simulink model "MiniDAQ_FOSWEC_V3_Sim"  (R2020b)
settings: Solver=FixedStepAuto  StartTime=0.0  StopTime=inf  FixedStep=0.01  RelTol=1e-3
libraries: slrealtimeethercatlib x12
settings Model: SimulationMode=external  Creator=Bret  LastModifiedBy=Bret
settings SolverCC: ConcurrentTasks=on  PositivePriorityOrder=on
settings OptimizationCC: BlockReduction=off  OptimizeBlockIOStorage=off
settings HardwareCC: ProdBitPerLong=64  ProdLongLongMode=on  ProdHWDeviceType=Intel->x86-64 (Linux 64)
settings RTWCC: Description=Simulink Real-Time  SystemTargetFile=slrealtime.tlc  TemplateMakefile=slrealtime_default_tmf  Toolchain=Simulink Real-Time Toolchain  BuildConfiguration=Faster Runs  CodeExecutionProfiling=on  TargetLang=C++

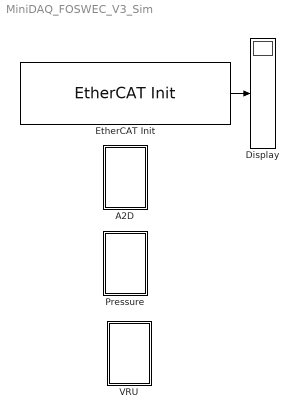
== system MiniDAQ_FOSWEC_V3_Sim ==
  A2D : Subsystem
  Display : Display
  EtherCAT Init : slrealtimeethercatlib/EtherCAT Init  Priority=0  config_file=C:\Users\Bret\Desktop\MiniDAQ_FOSWEC_V3\TwinCAT\MiniDAQ_V3.xml  device_id=0  pci_bus=0  pci_slot=0  pci_function=0  portnum=1  initstate=2  dctuning=0  enaDebug=0  enaDC=on  errLink=off  masterDbg=off  stateChgDbg=off  baseClock=off  masterCfg=off  logFile='c:\dbglog.txt'  sample_time=0.010000  DCMode=0
      settings: SourceProductBaseCode=XP
  Pressure : Subsystem
  VRU : Subsystem
  wires:
  EtherCAT Init/1 -> Display/1

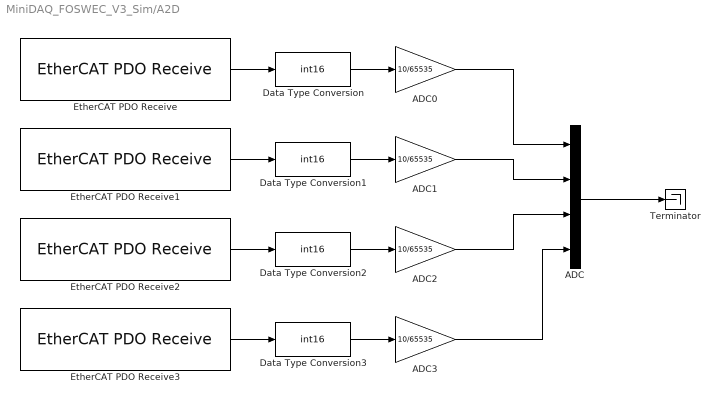
== system MiniDAQ_FOSWEC_V3_Sim/A2D ==
  ADC : Mux
  ADC{0..3} (4 alike) : Gain  Gain=10/65535
  Data Type Conversion{,1..3} (4 alike) : DataTypeConversion  OutDataTypeStr=int16
  EtherCAT PDO Receive : slrealtimeethercatlib/EtherCAT PDO Receive  Priority=2  sig_name=Box 1 (MiniDAQ_FOSWEC_V3).Inputs.ADC0  sig_offset=448  sig_type=uint16  type_size=16  sig_dim=1  device_id=0  sample_time=0.010000
      settings: SourceProductBaseCode=XP
  EtherCAT PDO Receive1 : slrealtimeethercatlib/EtherCAT PDO Receive  Priority=2  sig_name=Box 1 (MiniDAQ_FOSWEC_V3).Inputs.ADC1  sig_offset=464  sig_type=uint16  type_size=16  sig_dim=1  device_id=0  sample_time=0.010000
      settings: SourceProductBaseCode=XP
  EtherCAT PDO Receive2 : slrealtimeethercatlib/EtherCAT PDO Receive  Priority=2  sig_name=Box 1 (MiniDAQ_FOSWEC_V3).Inputs.ADC2  sig_offset=480  sig_type=uint16  type_size=16  sig_dim=1  device_id=0  sample_time=0.010000
      settings: SourceProductBaseCode=XP
  EtherCAT PDO Receive3 : slrealtimeethercatlib/EtherCAT PDO Receive  Priority=2  sig_name=Box 1 (MiniDAQ_FOSWEC_V3).Inputs.ADC3  sig_offset=432  sig_type=uint16  type_size=16  sig_dim=1  device_id=0  sample_time=0.010000
      settings: SourceProductBaseCode=XP
  Terminator : Terminator
  wires:
  ADC2/1 -> ADC/3
  ADC3/1 -> ADC/4
  Data Type Conversion2/1 -> ADC2/1
  EtherCAT PDO Receive3/1 -> Data Type Conversion3/1
  ADC/1 -> Terminator/1
  Data Type Conversion/1 -> ADC0/1
  ADC0/1 -> ADC/1
  ADC1/1 -> ADC/2
  EtherCAT PDO Receive/1 -> Data Type Conversion/1
  EtherCAT PDO Receive2/1 -> Data Type Conversion2/1
  Data Type Conversion3/1 -> ADC3/1
  Data Type Conversion1/1 -> ADC1/1
  EtherCAT PDO Receive1/1 -> Data Type Conversion1/1

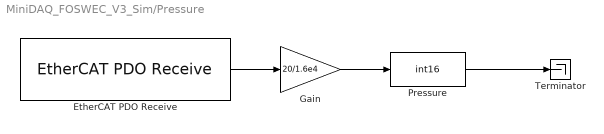
== system MiniDAQ_FOSWEC_V3_Sim/Pressure ==
  EtherCAT PDO Receive : slrealtimeethercatlib/EtherCAT PDO Receive  Priority=2  sig_name=Box 1 (MiniDAQ_FOSWEC_V3).Inputs.current0  sig_offset=496  sig_type=int16  type_size=16  sig_dim=1  device_id=0  sample_time=0.010000
      settings: SourceProductBaseCode=XP
  Gain : Gain  Gain=20/1.6e4
  Pressure : DataTypeConversion  OutDataTypeStr=int16
  Terminator : Terminator
  wires:
  Pressure/1 -> Terminator/1
  Gain/1 -> Pressure/1
  EtherCAT PDO Receive/1 -> Gain/1

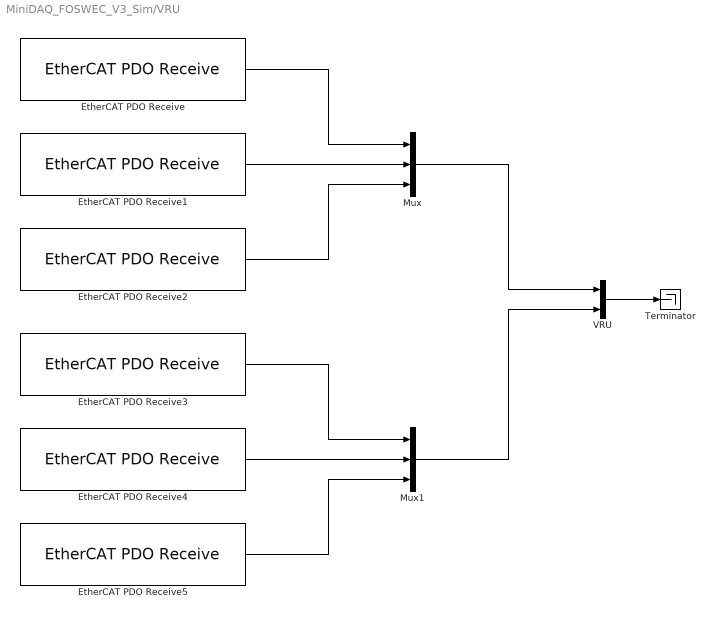
== system MiniDAQ_FOSWEC_V3_Sim/VRU ==
  EtherCAT PDO Receive : slrealtimeethercatlib/EtherCAT PDO Receive  Priority=2  sig_name=Box 1 (MiniDAQ_FOSWEC_V3).Inputs.acc_x  sig_offset=304  sig_type=single  type_size=32  sig_dim=1  device_id=0  sample_time=0.010000
      settings: SourceProductBaseCode=XP
  EtherCAT PDO Receive1 : slrealtimeethercatlib/EtherCAT PDO Receive  Priority=2  sig_name=Box 1 (MiniDAQ_FOSWEC_V3).Inputs.acc_y  sig_offset=336  sig_type=single  type_size=32  sig_dim=1  device_id=0  sample_time=0.010000
      settings: SourceProductBaseCode=XP
  EtherCAT PDO Receive2 : slrealtimeethercatlib/EtherCAT PDO Receive  Priority=2  sig_name=Box 1 (MiniDAQ_FOSWEC_V3).Inputs.acc_z  sig_offset=368  sig_type=single  type_size=32  sig_dim=1  device_id=0  sample_time=0.010000
      settings: SourceProductBaseCode=XP
  EtherCAT PDO Receive3 : slrealtimeethercatlib/EtherCAT PDO Receive  Priority=2  sig_name=Box 1 (MiniDAQ_FOSWEC_V3).Inputs.roll  sig_offset=208  sig_type=single  type_size=32  sig_dim=1  device_id=0  sample_time=0.010000
      settings: SourceProductBaseCode=XP
  EtherCAT PDO Receive4 : slrealtimeethercatlib/EtherCAT PDO Receive  Priority=2  sig_name=Box 1 (MiniDAQ_FOSWEC_V3).Inputs.pitch  sig_offset=240  sig_type=single  type_size=32  sig_dim=1  device_id=0  sample_time=0.010000
      settings: SourceProductBaseCode=XP
  EtherCAT PDO Receive5 : slrealtimeethercatlib/EtherCAT PDO Receive  Priority=2  sig_name=Box 1 (MiniDAQ_FOSWEC_V3).Inputs.yaw  sig_offset=272  sig_type=single  type_size=32  sig_dim=1  device_id=0  sample_time=0.010000
      settings: SourceProductBaseCode=XP
  Mux : Mux  Inputs=3
  Mux1 : Mux  Inputs=3
  Terminator : Terminator
  VRU : Mux  Inputs=2
  wires:
  EtherCAT PDO Receive1/1 -> Mux/2
  EtherCAT PDO Receive2/1 -> Mux/3
  EtherCAT PDO Receive/1 -> Mux/1
  Mux/1 -> VRU/1
  Mux1/1 -> VRU/2
  EtherCAT PDO Receive5/1 -> Mux1/3
  EtherCAT PDO Receive4/1 -> Mux1/2
  EtherCAT PDO Receive3/1 -> Mux1/1
  VRU/1 -> Terminator/1
